simulink model "BouncingBoxNoAttenuation"  (R2014b)
settings: Solver=ode45  StartTime=0.0  StopTime=100.0  RelTol=1e-3
libraries: vrlib x2
settings Model: Creator=Ben  LastModifiedBy=Ben

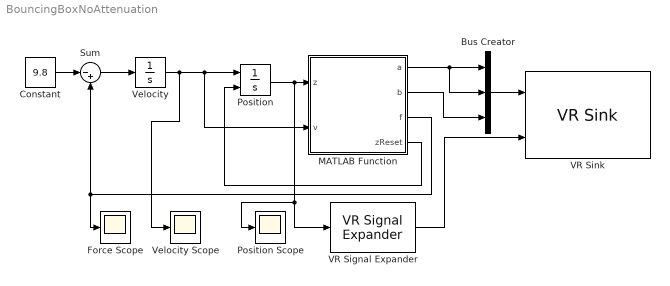
== system BouncingBoxNoAttenuation ==
  Bus Creator : BusCreator  Inputs=3
  Constant : Constant  Value=9.8
  Force Scope : Scope
      settings: TimeRange=100  YMin=0  YMax=400
  MATLAB Function : MATLAB Function  TreatAsAtomicUnit=on
  Position : Integrator  ExternalReset=rising  InitialCondition=15
  Position Scope : Scope
      settings: YMin=0  YMax=20
  Sum : Sum  Inputs=|-+
  VR Signal Expander : vrlib/VR Signal Expander  outwidth=3  outidx=[3]
  VR Sink : vrlib/VR Sink  InstantiateOnLoad=on  SampleTime=0.1  ViewEnable=on  RemoteChange=off  RemoteView=on  FieldsWritten=BoxTransform.scale.3.1.1.double#BoxTransform.translation.3.1.1.double  WorldFileName=BouncingBoxSimulink.wrl  WorldDescription=VRML scene BouncingBoxSimulink.wrl  AutoView=off  VideoDimensions=[]  AllowVariableSize=off  FigureProperties="{'Position', 'Name', 'Viewpoint', 'CameraBound', 'CameraDirection', 'CameraPosition', 'CameraUpVector', 'ZoomFactor', 'Antialiasing', 'Headlight', 'Lighting', 'NavPanel', 'Sound', 'StatusBar', 'Stereo3D', 'Stereo3DCameraOffset', 'Stereo3DHIT', 'ToolBar', 'Textures', 'Transparency', 'Triad', 'Wireframe', 'NavZones', 'NavMode', 'NavSpeed', 'CaptureFileFormat', 'CaptureFileName', 'Record2DCompressMethod', 'Record2DCompressQuality', 'Record2D', 'Record2DFileName', 'Record2DFPS'; [1.0500000000000000e+03   3.6100000000000000e+02   5.7600000000000000e+02   3.8000000000000000e+02], 'VRML scene BouncingBoxSimulink.wrl', 'Hello Matlab Simulink bouncing box!', 'on', [0.0000000000000000e+00   0.0000000000000000e+00  -1.0000000000000000e+00], [0.0000000000000000e+00   0.0000000000000000e+00   0.0000000000000000e+00], [0.0000000000000000e+00   1.0000000000000000e+00   0.0000000000000000e+00], [1.0000000000000000e+00], 'on', 'on', 'on', 'halfbar', 'on', 'on', 'off', [1.0000000149011612e-01], [0.0000000000000000e+00], 'on', 'on', 'on', 'none', 'off', 'off', 'walk', 'normal', 'tif', '%f_anim_%n.tif', 'auto', [7.5000000000000000e+01], 'off', '%f_anim_%n.avi', 'auto'}"
  Velocity : Integrator
  Velocity Scope : Scope
      settings: YMin=-20  YMax=20  SaveName=ScopeData2
  wires:
  MATLAB Function/3(f) -> Sum/2, Force Scope/1
  Constant/1 -> Sum/1
  Sum/1 -> Velocity/1
  VR Signal Expander/1 -> VR Sink/2
  MATLAB Function/1(a) -> Bus Creator/2, Bus Creator/1
  Bus Creator/1 -> VR Sink/1
  MATLAB Function/2(b) -> Bus Creator/3
  MATLAB Function/4(zReset) -> Position/2
  Position/1 -> Position Scope/1, VR Signal Expander/1, MATLAB Function/1(z)
  Velocity/1 -> MATLAB Function/2(v), Position/1, Velocity Scope/1

== matlab function BouncingBoxNoAttenuation/MATLAB Function ==
  data: a output; b output; z input; f output; v input; zReset output
% First edition date: Oct/10/2014
% Matlab 2014b Simulink VRtool
% Referance:http://www.mathworks.com/help/sl3d/examples/bouncing-ball.html"
% Revised date: Oct/17/2014
% 

function [a, b,f, zReset] = fcn(z, v)
%#codegen
f2=0;
zReset=0;   % Z position Reset signal =0 --> No reset

% Do not let z goes to negtive
if z<1e-4
    z=1e-4;
end

if z<1.5  % during compression
    f1=500*(1.5-z); % spring compression equations
    a=sqrt(1.5^3/z);
    b=z;
else      % during free fall
    f1=0;
    a=1.5;
    b=1.5;    
end 
f=f1+f2; % accumulated force
